simulink model "Two_models"  (R2021a)
settings: Solver=VariableStepAuto  StartTime=0.0  StopTime=1  FixedStep=0.01  RelTol=1e-3
libraries: simulink x6

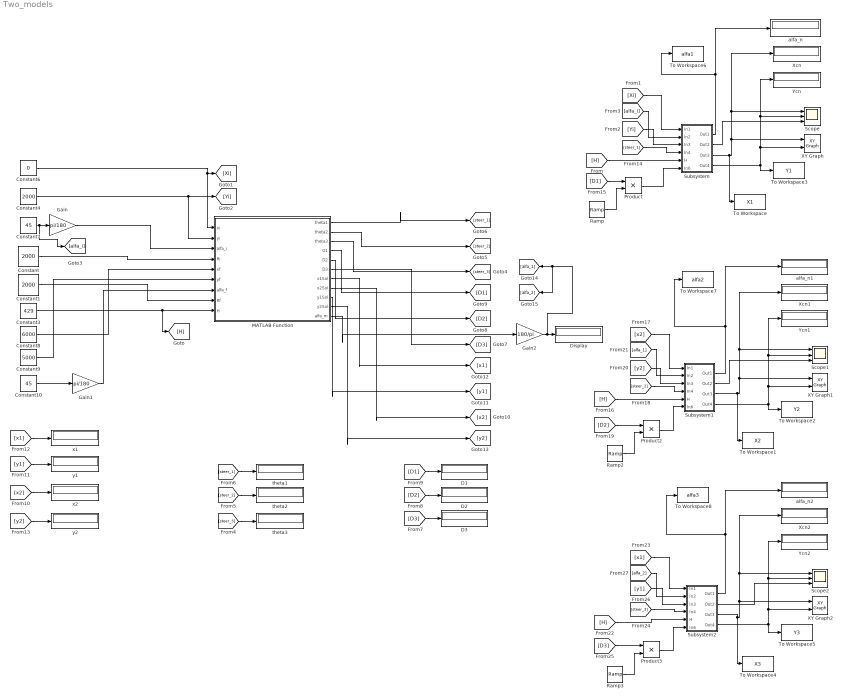
== system Two_models ==
  Constant : Constant  Value=2000
  Constant1 : Constant  Value=2000
  Constant10 : Constant  Value=45
  Constant3 : Constant  Value=429
  Constant4 : Constant  Value=2000
  Constant6 : Constant  Value=0
  Constant7 : Constant  Value=45
  Constant8 : Constant  Value=6000
  Constant9 : Constant  Value=5000
  D1 : Display
  D2 : Display
  D3 : Display
  Display : Display
  Gain : Gain  Gain=pi/180
  Gain1 : Gain  Gain=pi/180
  Gain2 : Gain  Gain=180/pi
  MATLAB Function : MATLAB Function  TreatAsAtomicUnit=on
  Product : Product
  Product2 : Product
  Product3 : Product
  Ramp : simulink/Sources/Ramp  slope=1  start=0  InitialOutput=0
  Ramp2 : simulink/Sources/Ramp  slope=1  start=0  InitialOutput=0
  Ramp3 : simulink/Sources/Ramp  slope=1  start=0  InitialOutput=0
  Scope : Scope  NumInputPorts=3
  Scope1 : Scope  NumInputPorts=3
  Scope2 : Scope  NumInputPorts=3
  Subsystem : Subsystem
  Subsystem1 : Subsystem
  Subsystem2 : Subsystem
  To Workspace : ToWorkspace  VariableName=X1  SampleTime=0.01
  To Workspace1 : ToWorkspace  VariableName=X2  SampleTime=0.01
  To Workspace2 : ToWorkspace  VariableName=Y2  SampleTime=0.01
  To Workspace3 : ToWorkspace  VariableName=Y1  SampleTime=0.01
  To Workspace4 : ToWorkspace  VariableName=X3  SampleTime=0.01
  To Workspace5 : ToWorkspace  VariableName=Y3  SampleTime=0.01
  To Workspace6 : ToWorkspace  VariableName=alfa1  SampleTime=0.01
  To Workspace7 : ToWorkspace  VariableName=alfa2  SampleTime=0.01
  To Workspace8 : ToWorkspace  VariableName=alfa3  SampleTime=0.01
  XY Graph : simulink/Sinks/XY Graph  xmin=-1000  xmax=5200  ymin=-1000  ymax=5200  st=0.01
  XY Graph1 : simulink/Sinks/XY Graph  xmin=-1000  xmax=5200  ymin=-1000  ymax=5200  st=0.01
  XY Graph2 : simulink/Sinks/XY Graph  xmin=-1000  xmax=5200  ymin=-1000  ymax=5200  st=0.01
  Xcn : Display
  Xcn1 : Display
  Xcn2 : Display
  Ycn : Display
  Ycn1 : Display
  Ycn2 : Display
  alfa_n : Display
  alfa_n1 : Display
  alfa_n2 : Display
  theta1 : Display
  theta2 : Display
  theta3 : Display
  x1 : Display
  x2 : Display
  y1 : Display
  y2 : Display
  wires:
  Subsystem/2(Out2) -> Scope/3
  [H] -> Subsystem/5(H)
  Subsystem/3(Out3) -> To Workspace/1, Xcn/1, Scope/1, XY Graph/1
  Constant6/1 -> [Xi], MATLAB Function/1(xi)
  MATLAB Function/1(theta1) -> [steer_1]
  Constant4/1 -> MATLAB Function/2(yi), [Yi]
  Subsystem/4(Out4) -> XY Graph/2, Ycn/1, Scope/2, To Workspace3/1
  Gain/1 -> MATLAB Function/3(alfa_i)
  MATLAB Function/6(D3) -> [D3]
  MATLAB Function/5(D2) -> [D2]
  MATLAB Function/7(x1Sol) -> [x1]
  MATLAB Function/8(x2Sol) -> [x2]
  Constant/1 -> MATLAB Function/4(Ri)
  MATLAB Function/10(y2Sol) -> [y2]
  Gain1/1 -> MATLAB Function/7(alfa_f)
  Constant9/1 -> MATLAB Function/6(yf)
  Constant7/1 -> [alfa_i], Gain/1
  MATLAB Function/9(y1Sol) -> [y1]
  Constant8/1 -> MATLAB Function/5(xf)
  MATLAB Function/4(D1) -> [D1]
  MATLAB Function/2(theta2) -> [steer_2]
  Constant3/1 -> [H], MATLAB Function/9(H)
  MATLAB Function/3(theta3) -> [steer_3]
  Constant10/1 -> Gain1/1
  Product/1 -> Subsystem/6(In6)
  [Xi] -> Subsystem/1(In1)
  [Yi] -> Subsystem/3(In3)
  [alfa_i] -> Subsystem/2(In2)
  [x1] -> x1/1
  [y1] -> y1/1
  [x2] -> x2/1
  [y2] -> y2/1
  [steer_1] -> Subsystem/4(In4)
  [D1] -> Product/1
  [D3] -> D3/1
  [steer_1] -> theta1/1
  [D2] -> D2/1
  [steer_2] -> theta2/1
  [D1] -> D1/1
  [steer_3] -> theta3/1
  [y2] -> Subsystem1/3(In3)
  [alfa_1] -> Subsystem1/2(In2)
  Subsystem1/1(Out1) -> To Workspace7/1, alfa_n1/1
  Subsystem1/3(Out3) -> To Workspace1/1, Xcn1/1, Scope1/1, XY Graph1/1
  Subsystem1/2(Out2) -> Scope1/3
  [x2] -> Subsystem1/1(In1)
  [D2] -> Product2/1
  [H] -> Subsystem1/5(H)
  Subsystem1/4(Out4) -> XY Graph1/2, Ycn1/1, Scope1/2, To Workspace2/1
  Product2/1 -> Subsystem1/6(In6)
  [steer_2] -> Subsystem1/4(In4)
  [y1] -> Subsystem2/3(In3)
  [alfa_2] -> Subsystem2/2(In2)
  Subsystem2/1(Out1) -> To Workspace8/1, alfa_n2/1
  Subsystem2/3(Out3) -> To Workspace4/1, Xcn2/1, Scope2/1, XY Graph2/1
  Subsystem2/2(Out2) -> Scope2/3
  [x1] -> Subsystem2/1(In1)
  [D3] -> Product3/1
  [H] -> Subsystem2/5(H)
  Subsystem2/4(Out4) -> To Workspace5/1, XY Graph2/2, Ycn2/1, Scope2/2
  Product3/1 -> Subsystem2/6(In6)
  [steer_3] -> Subsystem2/4(In4)
  Subsystem/1(Out1) -> To Workspace6/1, alfa_n/1
  Gain2/1 -> [alfa_2], [alfa_1], Display/1
  MATLAB Function/11(alfa_m) -> Gain2/1
  Constant1/1 -> MATLAB Function/8(Rf)
  Ramp/1 -> Product/2
  Ramp2/1 -> Product2/2
  Ramp3/1 -> Product3/2

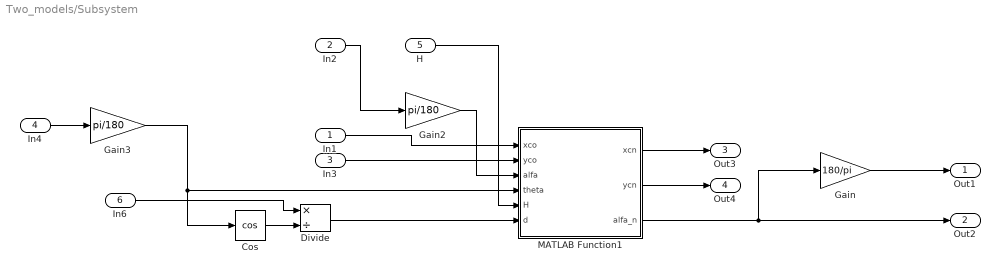
== system Two_models/Subsystem ==
  In1 : Inport
  In2 : Inport  Port=2
  In3 : Inport  Port=3
  In4 : Inport  Port=4
  H : Inport  Port=5
  In6 : Inport  Port=6
  Cos : Trigonometry  Operator=cos
  Divide : Product  Inputs=*/
  Gain : Gain  Gain=180/pi
  Gain2 : Gain  Gain=pi/180
  Gain3 : Gain  Gain=pi/180
  MATLAB Function1 : MATLAB Function  TreatAsAtomicUnit=on
  Out1 : Outport  VectorParamsAs1DForOutWhenUnconnected=off
  Out2 : Outport  Port=2  VectorParamsAs1DForOutWhenUnconnected=off
  Out3 : Outport  Port=3  VectorParamsAs1DForOutWhenUnconnected=off
  Out4 : Outport  Port=4  VectorParamsAs1DForOutWhenUnconnected=off
  wires:
  Gain2/1 -> MATLAB Function1/3(alfa)
  Divide/1 -> MATLAB Function1/6(d)
  In1/1 -> MATLAB Function1/1(xco)
  Gain/1 -> Out1/1
  Cos/1 -> Divide/2
  MATLAB Function1/3(alfa_n) -> Out2/1, Gain/1
  MATLAB Function1/2(ycn) -> Out4/1
  MATLAB Function1/1(xcn) -> Out3/1
  In6/1 -> Divide/1
  In3/1 -> MATLAB Function1/2(yco)
  Gain3/1 -> MATLAB Function1/4(theta), Cos/1
  H/1 -> MATLAB Function1/5(H)
  In2/1 -> Gain2/1
  In4/1 -> Gain3/1

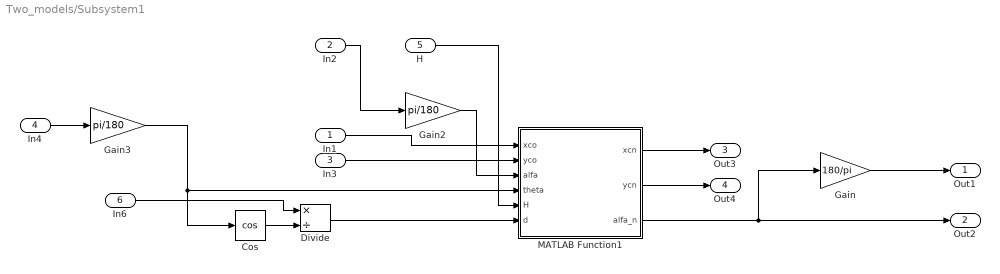
== system Two_models/Subsystem1 ==
  In1 : Inport
  In2 : Inport  Port=2
  In3 : Inport  Port=3
  In4 : Inport  Port=4
  H : Inport  Port=5
  In6 : Inport  Port=6
  Cos : Trigonometry  Operator=cos
  Divide : Product  Inputs=*/
  Gain : Gain  Gain=180/pi
  Gain2 : Gain  Gain=pi/180
  Gain3 : Gain  Gain=pi/180
  MATLAB Function1 : MATLAB Function  TreatAsAtomicUnit=on
  Out1 : Outport  VectorParamsAs1DForOutWhenUnconnected=off
  Out2 : Outport  Port=2  VectorParamsAs1DForOutWhenUnconnected=off
  Out3 : Outport  Port=3  VectorParamsAs1DForOutWhenUnconnected=off
  Out4 : Outport  Port=4  VectorParamsAs1DForOutWhenUnconnected=off
  wires:
  Gain2/1 -> MATLAB Function1/3(alfa)
  Divide/1 -> MATLAB Function1/6(d)
  In1/1 -> MATLAB Function1/1(xco)
  Gain/1 -> Out1/1
  Cos/1 -> Divide/2
  MATLAB Function1/3(alfa_n) -> Out2/1, Gain/1
  MATLAB Function1/2(ycn) -> Out4/1
  MATLAB Function1/1(xcn) -> Out3/1
  In6/1 -> Divide/1
  In3/1 -> MATLAB Function1/2(yco)
  Gain3/1 -> MATLAB Function1/4(theta), Cos/1
  H/1 -> MATLAB Function1/5(H)
  In2/1 -> Gain2/1
  In4/1 -> Gain3/1

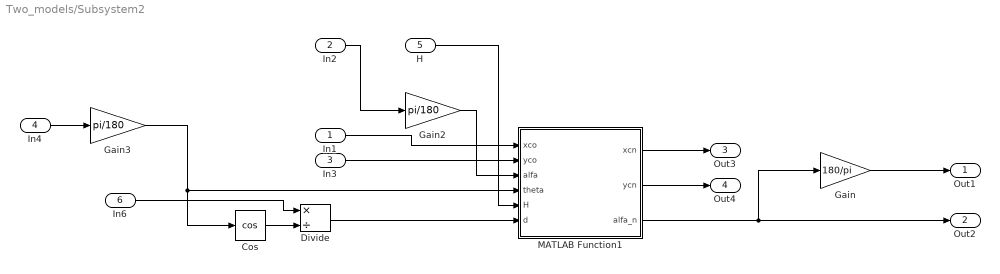
== system Two_models/Subsystem2 ==
  In1 : Inport
  In2 : Inport  Port=2
  In3 : Inport  Port=3
  In4 : Inport  Port=4
  H : Inport  Port=5
  In6 : Inport  Port=6
  Cos : Trigonometry  Operator=cos
  Divide : Product  Inputs=*/
  Gain : Gain  Gain=180/pi
  Gain2 : Gain  Gain=pi/180
  Gain3 : Gain  Gain=pi/180
  MATLAB Function1 : MATLAB Function  TreatAsAtomicUnit=on
  Out1 : Outport  VectorParamsAs1DForOutWhenUnconnected=off
  Out2 : Outport  Port=2  VectorParamsAs1DForOutWhenUnconnected=off
  Out3 : Outport  Port=3  VectorParamsAs1DForOutWhenUnconnected=off
  Out4 : Outport  Port=4  VectorParamsAs1DForOutWhenUnconnected=off
  wires:
  Cos/1 -> Divide/2
  Gain3/1 -> MATLAB Function1/4(theta), Cos/1
  In4/1 -> Gain3/1
  MATLAB Function1/3(alfa_n) -> Out2/1, Gain/1
  Divide/1 -> MATLAB Function1/6(d)
  H/1 -> MATLAB Function1/5(H)
  Gain2/1 -> MATLAB Function1/3(alfa)
  In6/1 -> Divide/1
  In2/1 -> Gain2/1
  MATLAB Function1/1(xcn) -> Out3/1
  MATLAB Function1/2(ycn) -> Out4/1
  In3/1 -> MATLAB Function1/2(yco)
  Gain/1 -> Out1/1
  In1/1 -> MATLAB Function1/1(xco)

== matlab function Two_models/Subsystem/MATLAB Function1 ==
function [xcn,ycn,alfa_n] = fcn(xco,yco,alfa,theta,H,d)
L=-H/cos((pi/2)-theta);
beta = d/L;
R = H *tan((pi/2)-theta);
gama = (((pi-beta)/2)-(alfa-pi/2));
alfa_n =(pi/2)+((alfa-pi/2)+beta) ;
xcn=xco+2*R*sin(beta/2)*cos(gama);
ycn=yco-2*R*sin(beta/2)*sin(gama);

== matlab function Two_models/Subsystem1/MATLAB Function1 ==
function [xcn,ycn,alfa_n] = fcn(xco,yco,alfa,theta,H,d)
L=-H/cos((pi/2)-theta);
beta = d/L;
R = H *tan((pi/2)-theta);
gama = (((pi-beta)/2)-(alfa-pi/2));
alfa_n =(pi/2)+((alfa-pi/2)+beta) ;
xcn=xco+2*R*sin(beta/2)*cos(gama);
ycn=yco-2*R*sin(beta/2)*sin(gama);

== matlab function Two_models/Subsystem2/MATLAB Function1 ==
function [xcn,ycn,alfa_n] = fcn(xco,yco,alfa,theta,H,d)
L=-H/cos((pi/2)-theta);
beta = d/L;
R = H *tan((pi/2)-theta);
gama = (((pi-beta)/2)-(alfa-pi/2));
alfa_n =(pi/2)+((alfa-pi/2)+beta) ;
xcn=xco+2*R*sin(beta/2)*cos(gama);
ycn=yco-2*R*sin(beta/2)*sin(gama);

== matlab function Two_models/MATLAB Function ==
function [theta1,theta2,theta3,D1,D2,D3,x1Sol,x2Sol,y1Sol,y2Sol,alfa_m] = fcn(xi,yi,alfa_i,Ri,xf,yf,alfa_f,Rf,H)


%H=200;
%Ri=500;Rf=500;
%xi=5000; yi=5000; alfa_i=90*pi/180;
%xf=0; yf=0; alfa_f=0*pi/180;


xc1=xf+Rf*sin(alfa_f-1e-10);
yc1=yf-Rf*cos(alfa_f-1e-10);
xc2=xi+Ri*sin(alfa_i-1e-10);
yc2=yi-Ri*cos(alfa_i-1e-10);

%v1=[(x1-xc1),(y1-yc1),0];
%v2=[(x1-x2),(y1-y2)],0;
%v3=[(x2-xc2),(y2-yc2),0];

%syms x1 y1 x2 y2 xc1 xc2 yc1 yc2 Rf Ri
%eqn1 = ((x1-xc1)*(x1-x2)+(y1-yc1)*(y1-y2)) == 0;
%eqn2 = ((x1 - xc1)*(y2 - yc2) - (x2 - xc2)*(y1 - yc1)) == 0;
%eqn3 = (x1-xc1)^2 + (y1-yc1)^2 == (Rf)^2;
%eqn4 = (x2-xc2)^2 + (y2-yc2)^2 == (Ri)^2;

%sol = solve([eqn1, eqn2, eqn3, eqn4], [x1, y1, x2, y2]);
%x1Sol = sol.x1
%y1Sol = sol.y1
%x2Sol = sol.x2
%y2Sol = sol.y2


x1Sol =(- Rf^2*Ri + Rf*Ri^2 - Rf*yc2^2 + yc1*Rf*yc2 + Ri*xc1^2 -xc2*Ri*xc1)/(Ri*(xc1 - xc2)) - ((Rf*yc1 - Rf*yc2)*(Ri^2*yc1 - Ri^2*yc2 + xc1^2*yc2 + xc2^2*yc2 - 2*yc1*yc2^2 + yc1^2*yc2 + yc2^3 + Ri*xc1*(- Rf^2 + 2*Rf*Ri - Ri^2 + xc1^2 - 2*xc1*xc2 + xc2^2 + yc1^2 - 2*yc1*yc2 + yc2^2)^(1/2) - Ri*xc2*(- Rf^2 + 2*Rf*Ri - Ri^2 + xc1^2 - 2*xc1*xc2 + xc2^2 + yc1^2 - 2*yc1*yc2 + yc2^2)^(1/2) - Rf*Ri*yc1 + Rf*Ri*yc2 - 2*xc1*xc2*yc2))/(Ri*(xc1 - xc2)*(xc1^2 - 2*xc1*xc2 + xc2^2 + yc1^2 - 2*yc1*yc2 + yc2^2));
 
%((Rf*yc1 - Rf*yc2)*(Ri^2*yc1 - Ri^2*yc2 + xc1^2*yc2 + xc2^2*yc2 - 2*yc1*yc2^2 + yc1^2*yc2 + yc2^3 + Ri*xc1*(- Rf^2 - 2*Rf*Ri - Ri^2 + xc1^2 - 2*xc1*xc2 + xc2^2 + yc1^2 - 2*yc1*yc2 + yc2^2)^(1/2) - Ri*xc2*(- Rf^2 - 2*Rf*Ri - Ri^2 + xc1^2 - 2*xc1*xc2 + xc2^2 + yc1^2 - 2*yc1*yc2 + yc2^2)^(1/2) + Rf*Ri*yc1 - Rf*Ri*yc2 - 2*xc1*xc2*yc2))/(Ri*(xc1 - xc2)*(xc1^2 - 2*xc1*xc2 + xc2^2 + yc1^2 - 2*yc1*yc2 + yc2^2)) - (Rf^2*Ri + Rf*Ri^2 - Rf*yc2^2 + yc1*Rf*yc2 - Ri*xc1^2 + xc2*Ri*xc1)/(Ri*(xc1 - xc2));
  
% ((Rf*yc1 - Rf*yc2)*(Ri^2*yc1 - Ri^2*yc2 + xc1^2*yc2 + xc2^2*yc2 - 2*yc1*yc2^2 + yc1^2*yc2 + yc2^3 - Ri*xc1*(- Rf^2 - 2*Rf*Ri - Ri^2 + xc1^2 - 2*xc1*xc2 + xc2^2 + yc1^2 - 2*yc1*yc2 + yc2^2)^(1/2) + Ri*xc2*(- Rf^2 - 2*Rf*Ri - Ri^2 + xc1^2 - 2*xc1*xc2 + xc2^2 + yc1^2 - 2*yc1*yc2 + yc2^2)^(1/2) + Rf*Ri*yc1 - Rf*Ri*yc2 - 2*xc1*xc2*yc2))/(Ri*(xc1 - xc2)*(xc1^2 - 2*xc1*xc2 + xc2^2 + yc1^2 - 2*yc1*yc2 + yc2^2)) - (Rf^2*Ri + Rf*Ri^2 - Rf*yc2^2 + yc1*Rf*yc2 - Ri*xc1^2 + xc2*Ri*xc1)/(Ri*(xc1 - xc2));
 
%(- Rf^2*Ri + Rf*Ri^2 - Rf*yc2^2 + yc1*Rf*yc2 + Ri*xc1^2 -xc2*Ri*xc1)/(Ri*(xc1 - xc2)) - ((Rf*yc1 - Rf*yc2)*(Ri^2*yc1 - Ri^2*yc2 + xc1^2*yc2 + xc2^2*yc2 - 2*yc1*yc2^2 + yc1^2*yc2 + yc2^3 + Ri*xc1*(- Rf^2 + 2*Rf*Ri - Ri^2 + xc1^2 - 2*xc1*xc2 + xc2^2 + yc1^2 - 2*yc1*yc2 + yc2^2)^(1/2) - Ri*xc2*(- Rf^2 + 2*Rf*Ri - Ri^2 + xc1^2 - 2*xc1*xc2 + xc2^2 + yc1^2 - 2*yc1*yc2 + yc2^2)^(1/2) - Rf*Ri*yc1 + Rf*Ri*yc2 - 2*xc1*xc2*yc2))/(Ri*(xc1 - xc2)*(xc1^2 - 2*xc1*xc2 + xc2^2 + yc1^2 - 2*yc1*yc2 + yc2^2));
 
%(- Rf^2*Ri + Rf*Ri^2 - Rf*yc2^2 + yc1*Rf*yc2 + Ri*xc1^2 -xc2*Ri*xc1)/(Ri*(xc1 - xc2)) - ((Rf*yc1 - Rf*yc2)*(Ri^2*yc1 - Ri^2*yc2 + xc1^2*yc2 + xc2^2*yc2 - 2*yc1*yc2^2 + yc1^2*yc2 + yc2^3 - Ri*xc1*(- Rf^2 + 2*Rf*Ri - Ri^2 + xc1^2 - 2*xc1*xc2 + xc2^2 + yc1^2 - 2*yc1*yc2 + yc2^2)^(1/2) + Ri*xc2*(- Rf^2 + 2*Rf*Ri - Ri^2 + xc1^2 - 2*xc1*xc2 + xc2^2 + yc1^2 - 2*yc1*yc2 + yc2^2)^(1/2) - Rf*Ri*yc1 + Rf*Ri*yc2 - 2*xc1*xc2*yc2))/(Ri*(xc1 - xc2)*(xc1^2 - 2*xc1*xc2 + xc2^2 + yc1^2 - 2*yc1*yc2 + yc2^2));
 
 
y1Sol =(Ri*yc1 - Rf*yc2 + (Rf*(Ri^2*yc1 - Ri^2*yc2 + xc1^2*yc2 + xc2^2*yc2 -2*yc1*yc2^2 + yc1^2*yc2 + yc2^3 + Ri*xc1*(- Rf^2 + 2*Rf*Ri - Ri^2 + xc1^2 - 2*xc1*xc2 + xc2^2 + yc1^2 - 2*yc1*yc2 + yc2^2)^(1/2) - Ri*xc2*(- Rf^2 + 2*Rf*Ri - Ri^2 + xc1^2 - 2*xc1*xc2 + xc2^2 + yc1^2 - 2*yc1*yc2 + yc2^2)^(1/2) - Rf*Ri*yc1 + Rf*Ri*yc2 - 2*xc1*xc2*yc2))/(xc1^2 - 2*xc1*xc2 + xc2^2 + yc1^2 - 2*yc1*yc2 + yc2^2))/Ri;


%(Rf*yc2 + Ri*yc1 - (Rf*(Ri^2*yc1 - Ri^2*yc2 + xc1^2*yc2 + xc2^2*yc2 - 2*yc1*yc2^2 + yc1^2*yc2 + yc2^3 + Ri*xc1*(- Rf^2 - 2*Rf*Ri - Ri^2 + xc1^2 - 2*xc1*xc2 + xc2^2 + yc1^2 - 2*yc1*yc2 + yc2^2)^(1/2) - Ri*xc2*(- Rf^2 - 2*Rf*Ri - Ri^2 + xc1^2 - 2*xc1*xc2 + xc2^2 + yc1^2 - 2*yc1*yc2 + yc2^2)^(1/2) + Rf*Ri*yc1 - Rf*Ri*yc2 - 2*xc1*xc2*yc2))/(xc1^2 - 2*xc1*xc2 + xc2^2 + yc1^2 - 2*yc1*yc2 + yc2^2))/Ri;

%(Rf*yc2 + Ri*yc1 - (Rf*(Ri^2*yc1 - Ri^2*yc2 + xc1^2*yc2 + xc2^2*yc2 -2*yc1*yc2^2 + yc1^2*yc2 + yc2^3 - Ri*xc1*(- Rf^2 - 2*Rf*Ri - Ri^2 + xc1^2 - 2*xc1*xc2 + xc2^2 + yc1^2 - 2*yc1*yc2 + yc2^2)^(1/2) + Ri*xc2*(- Rf^2 - 2*Rf*Ri - Ri^2 + xc1^2 - 2*xc1*xc2 + xc2^2 + yc1^2 - 2*yc1*yc2 + yc2^2)^(1/2) + Rf*Ri*yc1 - Rf*Ri*yc2 - 2*xc1*xc2*yc2))/(xc1^2 - 2*xc1*xc2 + xc2^2 + yc1^2 - 2*yc1*yc2 + yc2^2))/Ri;

%(Ri*yc1 - Rf*yc2 + (Rf*(Ri^2*yc1 - Ri^2*yc2 + xc1^2*yc2 + xc2^2*yc2 -2*yc1*yc2^2 + yc1^2*yc2 + yc2^3 + Ri*xc1*(- Rf^2 + 2*Rf*Ri - Ri^2 + xc1^2 - 2*xc1*xc2 + xc2^2 + yc1^2 - 2*yc1*yc2 + yc2^2)^(1/2) - Ri*xc2*(- Rf^2 + 2*Rf*Ri - Ri^2 + xc1^2 - 2*xc1*xc2 + xc2^2 + yc1^2 - 2*yc1*yc2 + yc2^2)^(1/2) - Rf*Ri*yc1 + Rf*Ri*yc2 - 2*xc1*xc2*yc2))/(xc1^2 - 2*xc1*xc2 + xc2^2 + yc1^2 - 2*yc1*yc2 + yc2^2))/Ri;
 
%(Ri*yc1 - Rf*yc2 + (Rf*(Ri^2*yc1 - Ri^2*yc2 + xc1^2*yc2 + xc2^2*yc2 -2*yc1*yc2^2 + yc1^2*yc2 + yc2^3 - Ri*xc1*(- Rf^2 + 2*Rf*Ri - Ri^2 + xc1^2 - 2*xc1*xc2 + xc2^2 + yc1^2 - 2*yc1*yc2 + yc2^2)^(1/2) + Ri*xc2*(- Rf^2 + 2*Rf*Ri - Ri^2 + xc1^2 - 2*xc1*xc2 + xc2^2 + yc1^2 - 2*yc1*yc2 + yc2^2)^(1/2) - Rf*Ri*yc1 + Rf*Ri*yc2 - 2*xc1*xc2*yc2))/(xc1^2 - 2*xc1*xc2 + xc2^2 + yc1^2 - 2*yc1*yc2 + yc2^2))/Ri;
 
 
x2Sol = - (- Ri^2 + Rf*Ri + xc2^2 - xc1*xc2 + yc2^2 - yc1*yc2)/(xc1 - xc2) - ((yc1 - yc2)*(Ri^2*yc1 - Ri^2*yc2 + xc1^2*yc2 + xc2^2*yc2 - 2*yc1*yc2^2 + yc1^2*yc2 + yc2^3 + Ri*xc1*(- Rf^2 + 2*Rf*Ri - Ri^2 + xc1^2 - 2*xc1*xc2 + xc2^2 + yc1^2 - 2*yc1*yc2 + yc2^2)^(1/2) - Ri*xc2*(- Rf^2 + 2*Rf*Ri - Ri^2 + xc1^2 - 2*xc1*xc2 + xc2^2 + yc1^2 - 2*yc1*yc2 + yc2^2)^(1/2) - Rf*Ri*yc1 + Rf*Ri*yc2 - 2*xc1*xc2*yc2))/((xc1 - xc2)*(xc1^2 - 2*xc1*xc2 + xc2^2 + yc1^2 - 2*yc1*yc2 + yc2^2));

% (Ri^2 + Rf*Ri - xc2^2 + xc1*xc2 - yc2^2 + yc1*yc2)/(xc1 - xc2) - ((yc1 - yc2)*(Ri^2*yc1 - Ri^2*yc2 + xc1^2*yc2 + xc2^2*yc2 - 2*yc1*yc2^2 + yc1^2*yc2 + yc2^3 + Ri*xc1*(- Rf^2 - 2*Rf*Ri - Ri^2 + xc1^2 - 2*xc1*xc2 + xc2^2 + yc1^2 - 2*yc1*yc2 + yc2^2)^(1/2) - Ri*xc2*(- Rf^2 - 2*Rf*Ri - Ri^2 + xc1^2 - 2*xc1*xc2 + xc2^2 + yc1^2 - 2*yc1*yc2 + yc2^2)^(1/2) + Rf*Ri*yc1 - Rf*Ri*yc2 - 2*xc1*xc2*yc2))/((xc1 - xc2)*(xc1^2 - 2*xc1*xc2 + xc2^2 + yc1^2 - 2*yc1*yc2 + yc2^2));
  
% (Ri^2 + Rf*Ri - xc2^2 + xc1*xc2 - yc2^2 + yc1*yc2)/(xc1 - xc2) - ((yc1 - yc2)*(Ri^2*yc1 - Ri^2*yc2 + xc1^2*yc2 + xc2^2*yc2 - 2*yc1*yc2^2 + yc1^2*yc2 + yc2^3 - Ri*xc1*(- Rf^2 - 2*Rf*Ri - Ri^2 + xc1^2 - 2*xc1*xc2 + xc2^2 + yc1^2 - 2*yc1*yc2 + yc2^2)^(1/2) + Ri*xc2*(- Rf^2 - 2*Rf*Ri - Ri^2 + xc1^2 - 2*xc1*xc2 + xc2^2 + yc1^2 - 2*yc1*yc2 + yc2^2)^(1/2) + Rf*Ri*yc1 - Rf*Ri*yc2 - 2*xc1*xc2*yc2))/((xc1 - xc2)*(xc1^2 - 2*xc1*xc2 + xc2^2 + yc1^2 - 2*yc1*yc2 + yc2^2));

% - (- Ri^2 + Rf*Ri + xc2^2 - xc1*xc2 + yc2^2 - yc1*yc2)/(xc1 - xc2) - ((yc1 - yc2)*(Ri^2*yc1 - Ri^2*yc2 + xc1^2*yc2 + xc2^2*yc2 - 2*yc1*yc2^2 + yc1^2*yc2 + yc2^3 + Ri*xc1*(- Rf^2 + 2*Rf*Ri - Ri^2 + xc1^2 - 2*xc1*xc2 + xc2^2 + yc1^2 - 2*yc1*yc2 + yc2^2)^(1/2) - Ri*xc2*(- Rf^2 + 2*Rf*Ri - Ri^2 + xc1^2 - 2*xc1*xc2 + xc2^2 + yc1^2 - 2*yc1*yc2 + yc2^2)^(1/2) - Rf*Ri*yc1 + Rf*Ri*yc2 - 2*xc1*xc2*yc2))/((xc1 - xc2)*(xc1^2 - 2*xc1*xc2 + xc2^2 + yc1^2 - 2*yc1*yc2 + yc2^2));

% - (- Ri^2 + Rf*Ri + xc2^2 - xc1*xc2 + yc2^2 - yc1*yc2)/(xc1 - xc2) - ((yc1 - yc2)*(Ri^2*yc1 - Ri^2*yc2 + xc1^2*yc2 + xc2^2*yc2 - 2*yc1*yc2^2 + yc1^2*yc2 + yc2^3 - Ri*xc1*(- Rf^2 + 2*Rf*Ri - Ri^2 + xc1^2 - 2*xc1*xc2 + xc2^2 + yc1^2 - 2*yc1*yc2 + yc2^2)^(1/2) + Ri*xc2*(- Rf^2 + 2*Rf*Ri - Ri^2 + xc1^2 - 2*xc1*xc2 + xc2^2 + yc1^2 - 2*yc1*yc2 + yc2^2)^(1/2) - Rf*Ri*yc1 + Rf*Ri*yc2 - 2*xc1*xc2*yc2))/((xc1 - xc2)*(xc1^2 - 2*xc1*xc2 + xc2^2 + yc1^2 - 2*yc1*yc2 + yc2^2));
 
 
y2Sol =(Ri^2*yc1 - Ri^2*yc2 + xc1^2*yc2 + xc2^2*yc2 - 2*yc1*yc2^2 + yc1^2*yc2 + yc2^3 + Ri*xc1*(- Rf^2 + 2*Rf*Ri - Ri^2 + xc1^2 - 2*xc1*xc2 + xc2^2 + yc1^2 - 2*yc1*yc2 + yc2^2)^(1/2) - Ri*xc2*(- Rf^2 + 2*Rf*Ri - Ri^2 + xc1^2 - 2*xc1*xc2 + xc2^2 + yc1^2 - 2*yc1*yc2 + yc2^2)^(1/2) - Rf*Ri*yc1 + Rf*Ri*yc2 - 2*xc1*xc2*yc2)/(xc1^2 - 2*xc1*xc2 + xc2^2 + yc1^2 - 2*yc1*yc2 + yc2^2);
 
%(Ri^2*yc1 - Ri^2*yc2 + xc1^2*yc2 + xc2^2*yc2 - 2*yc1*yc2^2 + yc1^2*yc2 + yc2^3 + Ri*xc1*(- Rf^2 - 2*Rf*Ri - Ri^2 + xc1^2 - 2*xc1*xc2 + xc2^2 + yc1^2 - 2*yc1*yc2 + yc2^2)^(1/2) - Ri*xc2*(- Rf^2 - 2*Rf*Ri - Ri^2 + xc1^2 - 2*xc1*xc2 + xc2^2 + yc1^2 - 2*yc1*yc2 + yc2^2)^(1/2) + Rf*Ri*yc1 - Rf*Ri*yc2 - 2*xc1*xc2*yc2)/(xc1^2 - 2*xc1*xc2 + xc2^2 + yc1^2 - 2*yc1*yc2 + yc2^2);
 
%(Ri^2*yc1 - Ri^2*yc2 + xc1^2*yc2 + xc2^2*yc2 - 2*yc1*yc2^2 + yc1^2*yc2 +yc2^3 - Ri*xc1*(- Rf^2 - 2*Rf*Ri - Ri^2 + xc1^2 - 2*xc1*xc2 + xc2^2 + yc1^2 - 2*yc1*yc2 + yc2^2)^(1/2) + Ri*xc2*(- Rf^2 - 2*Rf*Ri - Ri^2 + xc1^2 - 2*xc1*xc2 + xc2^2 + yc1^2 - 2*yc1*yc2 + yc2^2)^(1/2) + Rf*Ri*yc1 - Rf*Ri*yc2 - 2*xc1*xc2*yc2)/(xc1^2 - 2*xc1*xc2 + xc2^2 + yc1^2 - 2*yc1*yc2 + yc2^2);
 
%(Ri^2*yc1 - Ri^2*yc2 + xc1^2*yc2 + xc2^2*yc2 - 2*yc1*yc2^2 + yc1^2*yc2 + yc2^3 + Ri*xc1*(- Rf^2 + 2*Rf*Ri - Ri^2 + xc1^2 - 2*xc1*xc2 + xc2^2 + yc1^2 - 2*yc1*yc2 + yc2^2)^(1/2) - Ri*xc2*(- Rf^2 + 2*Rf*Ri - Ri^2 + xc1^2 - 2*xc1*xc2 + xc2^2 + yc1^2 - 2*yc1*yc2 + yc2^2)^(1/2) - Rf*Ri*yc1 + Rf*Ri*yc2 - 2*xc1*xc2*yc2)/(xc1^2 - 2*xc1*xc2 + xc2^2 + yc1^2 - 2*yc1*yc2 + yc2^2);
 
%(Ri^2*yc1 - Ri^2*yc2 + xc1^2*yc2 + xc2^2*yc2 - 2*yc1*yc2^2 + yc1^2*yc2 + yc2^3 - Ri*xc1*(- Rf^2 + 2*Rf*Ri - Ri^2 + xc1^2 - 2*xc1*xc2 + xc2^2 + yc1^2 - 2*yc1*yc2 + yc2^2)^(1/2) + Ri*xc2*(- Rf^2 + 2*Rf*Ri - Ri^2 + xc1^2 - 2*xc1*xc2 + xc2^2 + yc1^2 - 2*yc1*yc2 + yc2^2)^(1/2) - Rf*Ri*yc1 + Rf*Ri*yc2 - 2*xc1*xc2*yc2)/(xc1^2 - 2*xc1*xc2 + xc2^2 + yc1^2 - 2*yc1*yc2 + yc2^2);

d2x1=cos(alfa_i);
d2y1=sin(alfa_i);
d2x2=x2Sol-xi;
d2y2=y2Sol-yi;
Cross2=(d2x1*d2y2-d2y1*d2x2);

d1x1=cos(alfa_f);
d1y1=sin(alfa_f);
d1x2=x1Sol-xf;
d1y2=y1Sol-yf;
Cross1=(d1x1*d1y2-d1y1*d1x2);

if (Cross2 > 0)
   sign_1st=-1;
else  
    sign_1st=1;
end 

if (Cross1 > 0)
   sign_2nd=-1;
else  
    sign_2nd=1;
end 

theta1=sign_1st*(90-atand(Ri/H));
theta2=0.000001;
theta3=sign_2nd*(90-atand(Rf/H));

%sign_1st*(90-atand(Ri/H));
%sign_1st*
%sign_2nd*

cosangle1=((y2Sol-yi)*sin(alfa_i)+(x2Sol-xi)*cos(alfa_i));

if (cosangle1 < 0)
   s_1st=-1;
else  
    s_1st=1;
end 

D1=s_1st*Ri*acos((((x2Sol-xc2)*(xi-xc2)+(y2Sol-yc2)*(yi-yc2))/Ri^2)-9e-15);

L=-H/cos((pi/2)-theta1*pi/180);
beta = D1/(L*cos(theta1*pi/180));
alfa_m =  alfa_i + beta;

cosangle2=((y1Sol-y2Sol)*sin(alfa_m)+(x1Sol-x2Sol)*cos(alfa_m));
cosangle3=((yf-y1Sol)*sin(alfa_m)+(xf-x1Sol)*cos(alfa_m));

if (cosangle2 < 0)
   s_2nd=-1;
else  
    s_2nd=1;
end 
if (cosangle3 < 0)
   s_3rd=-1;
else  
    s_3rd=1;
end 



D2=s_2nd*((x1Sol-x2Sol)^2+(y1Sol-y2Sol)^2)^0.5;
D3=s_3rd*Rf*acos((((x1Sol-xc1)*(xf-xc1)+(y1Sol-yc1)*(yf-yc1))/Rf^2)-9e-15);

%s_1st*
%s_1st*s_2nd*
%s_1st*s_2nd*s_3rd*
